simulink model "closeLoop"  (R2024a)
settings: Solver=ode45  StartTime=0.0  StopTime=100  RelTol=1e-3
values from neighbouring files (symbols this model uses):
  x = [input(1);input(2);input(3)]    [Dist_observer.m]
  y = [input(4),input(5),input(6)]'    [controller.m]
undefined symbols (not defined in the file or in its folder): initial_1, observer, saturation, z
libraries: simulink x3, slpidlib x3
settings Model: Creator=b_ant  LastModifiedBy=b_ant
settings SolverCC: ZeroCrossAlgorithm=Adaptive
settings DebuggingCC: IgnoredZcDiagnostic=none

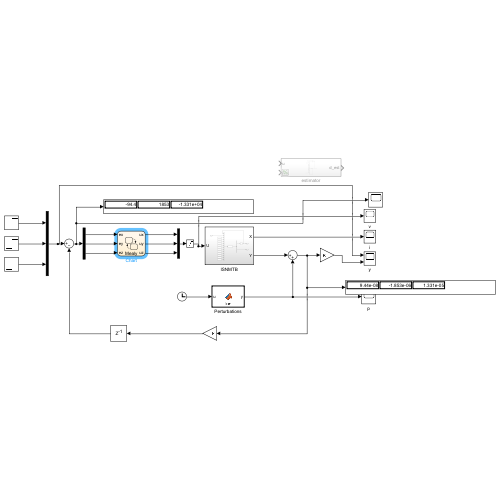
[thumbnail: Simulink's stored preview of the top-level diagram]
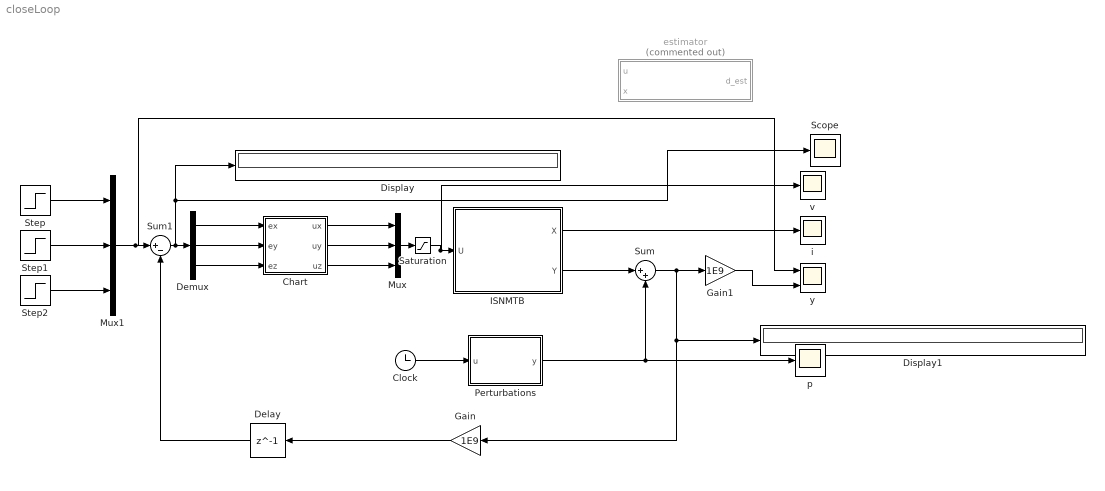
== system closeLoop ==
  Chart : Stateflow chart  TreatAsAtomicUnit=on
      settings: PortSchema="{\"entries\":[{\"content\":{\"sides\":[{\"content\":{\"connectorIds\":[\"In2\",\"In3\",\"In1\"]},\"type\":\"ConnectorPlacement.EquallySpacedRectSide\",\"uuid\":\"8b74e5db-fe86-432f-bb0a-8ff1b800d4e3\"},{\"content\":{\"connectorIds\":[\"Out2\",\"Out3\",\"Out1\"],\"side\":\"RIGHT\"},\"type\":\"ConnectorPlacement.EquallySpacedRectSide\",\"uuid\":\"0c774d5f-25b7-41fd-8d4f-dcece7db4dd0\"},{\"content\":{\"side\":\"TOP\"},\"type\":\"ConnectorPlacement.EquallySpacedRectSide\",\"uuid\":\"bb376f1f-a9bb-4d19-8a5b-9121a4c7bbab\"}]},\"type\":\"ConnectorPlacement.EquallySpacedConnector\",\"uuid\":\"4c5f25f9-8a94-4cb2-acc7-8586629943a0\"}],\"packageUris\":[\"http://schema.mathworks.com/mf0/Connector/R2020b\"],\"version\":\"1.0\"}"
  Clock : Clock
      settings: Decimation=1000
  Delay : Delay  DelayLength=1  InitialCondition=[3E4,-2E4,3E4]'  SampleTime=1E-6
  Demux : Demux  Outputs=3
  Display : Display
  Display1 : Display
  Gain : Gain  Gain=1E9
  Gain1 : Gain  Gain=1E9
  ISNMTB : Subsystem
  Mux : Mux  Inputs=3
  Mux1 : Mux  Inputs=3
  Perturbations : MATLAB Function  TreatAsAtomicUnit=on
  Saturation : Saturate  UpperLimit=[15,7,15]'  LowerLimit=[-15,-7,-15]'
  Scope : Scope
  Step : Step  After=0  SampleTime=0
  Step1 : Step  After=0  SampleTime=0
  Step2 : Step  After=0  SampleTime=0
  Sum : Sum  Inputs=|++
  Sum1 : Sum  Inputs=|+-
  estimator : Subsystem  Commented=on
  i : Scope
  p : Scope
  v : Scope
  y : Scope  NumInputPorts=2
  wires:
  ISNMTB/1(X) -> i/1
  Perturbations/1(y) -> p/1, Sum/2
  Clock/1 -> Perturbations/1(u)
  ISNMTB/2(Y) -> Sum/1
  Sum/1 -> Display1/1, Gain/1, Gain1/1
  Step/1 -> Mux1/1
  Step2/1 -> Mux1/3
  Step1/1 -> Mux1/2
  Mux1/1 -> y/1, Sum1/1
  Gain1/1 -> y/2
  Saturation/1 -> v/1, ISNMTB/1(U)
  Sum1/1 -> Scope/1, Display/1, Demux/1
  Mux/1 -> Saturation/1
  Demux/1 -> Chart/2(ex)
  Chart/2(ux) -> Mux/1
  Demux/2 -> Chart/3(ey)
  Demux/3 -> Chart/1(ez)
  Chart/1(uz) -> Mux/3
  Chart/3(uy) -> Mux/2
  Delay/1 -> Sum1/2
  Gain/1 -> Delay/1

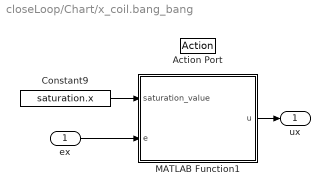
== system closeLoop/Chart/x_coil.bang_bang ==
  ex : Inport
  Action Port : ActionPort
      settings: CopyFcn=Stateflow.SLINSF.SimulinkMan.removeBlockPreDeleteFcn  PreDeleteFcn=Stateflow.SLINSF.SimulinkMan.unsafePredeleteFcn
  Constant9 : Constant  Value=saturation.x
  MATLAB Function1 : MATLAB Function  TreatAsAtomicUnit=on
  ux : Outport
  wires:
  MATLAB Function1/1(u) -> ux/1
  ex/1 -> MATLAB Function1/2(e)
  Constant9/1 -> MATLAB Function1/1(saturation_value)

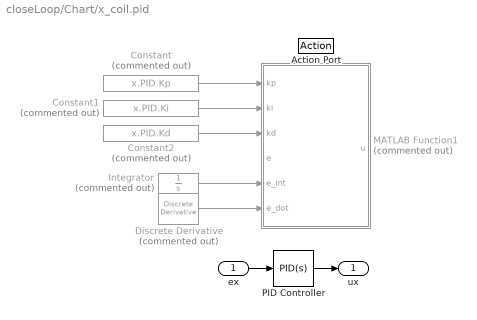
== system closeLoop/Chart/x_coil.pid ==
  ex : Inport
  Action Port : ActionPort
      settings: CopyFcn=Stateflow.SLINSF.SimulinkMan.removeBlockPreDeleteFcn  PreDeleteFcn=Stateflow.SLINSF.SimulinkMan.unsafePredeleteFcn
  Constant : Constant  Commented=on  Value=x.PID.Kp
  Constant1 : Constant  Commented=on  Value=x.PID.Ki
  Constant2 : Constant  Commented=on  Value=x.PID.Kd
  Discrete Derivative : simulink/Discrete/Discrete Derivative  Commented=on  gainval=1.0  ICPrevScaledInput=0.0  OutMin=[]  OutMax=[]  OutDataType=fixdt(1, 16)  OutScaling=2^-10  DoSatur=off
  Integrator : Integrator  Commented=on
  MATLAB Function1 : MATLAB Function  Commented=on  TreatAsAtomicUnit=on
  PID Controller : slpidlib/PID Controller  Controller=PID  Form=Parallel  TimeDomain=Continuous-time  UseExternalTs=off  SampleTime=-1  IntegratorMethod=Forward Euler  FilterMethod=Forward Euler  ControllerParametersSource=internal  P=x.PID.Kp  I=x.PID.Ki  UseKiTs=off  D=x.PID.Kd  UseExternalDerivativeSource=off  N=100  UseFilter=on  TunerSelectOption=Transfer Function Based (PID Tuner App)  InitialConditionSource=internal  InitialConditionForIntegrator=0  InitialConditionForFilter=0  DifferentiatorICPrevScaledInput=0  ExternalReset=none  TrackingMode=off  Kt=1  LimitOutput=off  SatLimitsSource=internal  UpperSaturationLimit=inf  LowerSaturationLimit=-inf  LinearizeAsGain=on  AntiWindupMode=none  Kb=1  LimitIntegrator=off  UpperIntegratorSaturationLimit=inf  LowerIntegratorSaturationLimit=-inf  POutMin=[]  POutMax=[]  IOutMin=[]  IOutMax=[]  DOutMin=[]  DOutMax=[]  NOutMin=[]  NOutMax=[]  SumOutMin=[]  SumOutMax=[]  SaturationOutMin=[]  SaturationOutMax=[]  PParamMin=[]  PParamMax=[]  IParamMin=[]  IParamMax=[]  DParamMin=[]  DParamMax=[]  NParamMin=[]  NParamMax=[]  KbParamMin=[]  KbParamMax=[]  KtParamMin=[]  KtParamMax=[]  KbOutMin=[]  KbOutMax=[]  KtOutMin=[]  KtOutMax=[]  IntegratorOutMin=[]  IntegratorOutMax=[]  FilterOutMin=[]  FilterOutMax=[]  SumI1OutMin=[]  SumI1OutMax=[]  SumI2OutMin=[]  SumI2OutMax=[]  SumI3OutMin=[]  SumI3OutMax=[]  SumI4OutMin=[]  SumI4OutMax=[]  SumDOutMin=[]  SumDOutMax=[]  DifferentiatorOutMin=[]  DifferentiatorOutMax=[]  FilterDiffOutCoefMin=[]  FilterDiffOutCoefMax=[]  ReciprocalOutMin=[]  ReciprocalOutMax=[]  SumDenOutMin=[]  SumDenOutMax=[]  SumNumOutMin=[]  SumNumOutMax=[]  DivideOutMin=[]  DivideOutMax=[]  UdiffTsProdOutMin=[]  UdiffTsProdOutMax=[]  NTsProdOutMin=[]  NTsProdOutMax=[]  UintegralTsProdOutMin=[]  UintegralTsProdOutMax=[]  UngainTsProdOutMin=[]  UngainTsProdOutMax=[]  ClampingZeroOutDataTypeStr=Inherit: Inherit via back propagation  ClampingZeroOutMin=[]  ClampingZeroOutMax=[]  FilterDenConstantOutDataTypeStr=Inherit: Inherit via back propagation  FilterDenConstantOutMin=[]  FilterDenConstantOutMax=[]  PCopyOutDataTypeStr=Inherit: Inherit via back propagation  PCopyOutMin=[]  PCopyOutMax=[]  NCopyOutDataTypeStr=Inherit: Inherit via back propagation  NCopyOutMin=[]  NCopyOutMax=[]  IntegratorContinuousStateAttributes=''  IntegratorStateMustResolveToSignalObject=off  IntegratorRTWStateStorageClass=Auto  FilterContinuousStateAttributes=''  FilterStateMustResolveToSignalObject=off  FilterRTWStateStorageClass=Auto  ParallelPVariant=InternalParameters  IdealPVariant=Disabled  IVariant=InternalParameters  DVariant=InternalParameters  IntegratorVariant=Continuous  SatVariant=Disabled  AWVariant=Passthrough  PCopyVariant=Disabled  TRVariant=Disabled  FdbkBlocksVariant=Forward  IdealPFdbkVariant=Disabled  SatFdbkVariant=Disabled  DerivativeFilterVariant=ContFilter  NVariant=InternalParameters  NCopyVariant=Disabled  FilterICVariant=InternalICsFilter  IntegratorICVariant=InternalICs  ExternalResetVariant=Disabled  TRSumVariant=Passthrough  SumFdbkVariant=Disabled  SumVariant=Sum_PID  TsampFilterVariant=InternalTs  TsampNgainVariant=Passthrough  TsampIntegralVariant=Disabled_SignalSpec  ExternalSaturationOutDataTypeStr=Inherit: Same as second input  DerivativeSourceVariant=ErrorSignal
  ux : Outport
  wires:
  Integrator/1 -> MATLAB Function1/5(e_int)
  Constant1/1 -> MATLAB Function1/2(ki)
  Constant2/1 -> MATLAB Function1/3(kd)
  Discrete Derivative/1 -> MATLAB Function1/6(e_dot)
  Constant/1 -> MATLAB Function1/1(kp)
  PID Controller/1 -> ux/1
  ex/1 -> PID Controller/1

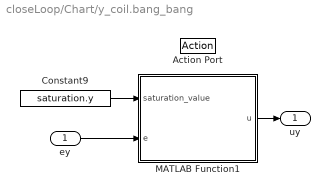
== system closeLoop/Chart/y_coil.bang_bang ==
  ey : Inport
  Action Port : ActionPort
      settings: CopyFcn=Stateflow.SLINSF.SimulinkMan.removeBlockPreDeleteFcn  PreDeleteFcn=Stateflow.SLINSF.SimulinkMan.unsafePredeleteFcn
  Constant9 : Constant  Value=saturation.y
  MATLAB Function1 : MATLAB Function  TreatAsAtomicUnit=on
  uy : Outport
  wires:
  MATLAB Function1/1(u) -> uy/1
  ey/1 -> MATLAB Function1/2(e)
  Constant9/1 -> MATLAB Function1/1(saturation_value)

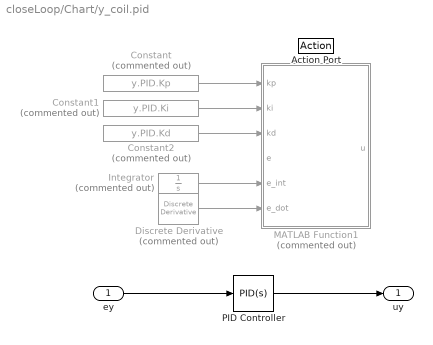
== system closeLoop/Chart/y_coil.pid ==
  ey : Inport
  Action Port : ActionPort
      settings: CopyFcn=Stateflow.SLINSF.SimulinkMan.removeBlockPreDeleteFcn  PreDeleteFcn=Stateflow.SLINSF.SimulinkMan.unsafePredeleteFcn
  Constant : Constant  Commented=on  Value=y.PID.Kp
  Constant1 : Constant  Commented=on  Value=y.PID.Ki
  Constant2 : Constant  Commented=on  Value=y.PID.Kd
  Discrete Derivative : simulink/Discrete/Discrete Derivative  Commented=on  gainval=1.0  ICPrevScaledInput=0.0  OutMin=[]  OutMax=[]  OutDataType=fixdt(1, 16)  OutScaling=2^-10  DoSatur=off
  Integrator : Integrator  Commented=on
  MATLAB Function1 : MATLAB Function  Commented=on  TreatAsAtomicUnit=on
  PID Controller : slpidlib/PID Controller  Controller=PID  Form=Parallel  TimeDomain=Continuous-time  UseExternalTs=off  SampleTime=-1  IntegratorMethod=Forward Euler  FilterMethod=Forward Euler  ControllerParametersSource=internal  P=y.PID.Kp  I=y.PID.Ki  UseKiTs=off  D=y.PID.Kd  UseExternalDerivativeSource=off  N=100  UseFilter=on  TunerSelectOption=Transfer Function Based (PID Tuner App)  InitialConditionSource=internal  InitialConditionForIntegrator=0  InitialConditionForFilter=0  DifferentiatorICPrevScaledInput=0  ExternalReset=none  TrackingMode=off  Kt=1  LimitOutput=off  SatLimitsSource=internal  UpperSaturationLimit=inf  LowerSaturationLimit=-inf  LinearizeAsGain=on  AntiWindupMode=none  Kb=1  LimitIntegrator=off  UpperIntegratorSaturationLimit=inf  LowerIntegratorSaturationLimit=-inf  POutMin=[]  POutMax=[]  IOutMin=[]  IOutMax=[]  DOutMin=[]  DOutMax=[]  NOutMin=[]  NOutMax=[]  SumOutMin=[]  SumOutMax=[]  SaturationOutMin=[]  SaturationOutMax=[]  PParamMin=[]  PParamMax=[]  IParamMin=[]  IParamMax=[]  DParamMin=[]  DParamMax=[]  NParamMin=[]  NParamMax=[]  KbParamMin=[]  KbParamMax=[]  KtParamMin=[]  KtParamMax=[]  KbOutMin=[]  KbOutMax=[]  KtOutMin=[]  KtOutMax=[]  IntegratorOutMin=[]  IntegratorOutMax=[]  FilterOutMin=[]  FilterOutMax=[]  SumI1OutMin=[]  SumI1OutMax=[]  SumI2OutMin=[]  SumI2OutMax=[]  SumI3OutMin=[]  SumI3OutMax=[]  SumI4OutMin=[]  SumI4OutMax=[]  SumDOutMin=[]  SumDOutMax=[]  DifferentiatorOutMin=[]  DifferentiatorOutMax=[]  FilterDiffOutCoefMin=[]  FilterDiffOutCoefMax=[]  ReciprocalOutMin=[]  ReciprocalOutMax=[]  SumDenOutMin=[]  SumDenOutMax=[]  SumNumOutMin=[]  SumNumOutMax=[]  DivideOutMin=[]  DivideOutMax=[]  UdiffTsProdOutMin=[]  UdiffTsProdOutMax=[]  NTsProdOutMin=[]  NTsProdOutMax=[]  UintegralTsProdOutMin=[]  UintegralTsProdOutMax=[]  UngainTsProdOutMin=[]  UngainTsProdOutMax=[]  ClampingZeroOutDataTypeStr=Inherit: Inherit via back propagation  ClampingZeroOutMin=[]  ClampingZeroOutMax=[]  FilterDenConstantOutDataTypeStr=Inherit: Inherit via back propagation  FilterDenConstantOutMin=[]  FilterDenConstantOutMax=[]  PCopyOutDataTypeStr=Inherit: Inherit via back propagation  PCopyOutMin=[]  PCopyOutMax=[]  NCopyOutDataTypeStr=Inherit: Inherit via back propagation  NCopyOutMin=[]  NCopyOutMax=[]  IntegratorContinuousStateAttributes=''  IntegratorStateMustResolveToSignalObject=off  IntegratorRTWStateStorageClass=Auto  FilterContinuousStateAttributes=''  FilterStateMustResolveToSignalObject=off  FilterRTWStateStorageClass=Auto  ParallelPVariant=InternalParameters  IdealPVariant=Disabled  IVariant=InternalParameters  DVariant=InternalParameters  IntegratorVariant=Continuous  SatVariant=Disabled  AWVariant=Passthrough  PCopyVariant=Disabled  TRVariant=Disabled  FdbkBlocksVariant=Forward  IdealPFdbkVariant=Disabled  SatFdbkVariant=Disabled  DerivativeFilterVariant=ContFilter  NVariant=InternalParameters  NCopyVariant=Disabled  FilterICVariant=InternalICsFilter  IntegratorICVariant=InternalICs  ExternalResetVariant=Disabled  TRSumVariant=Passthrough  SumFdbkVariant=Disabled  SumVariant=Sum_PID  TsampFilterVariant=InternalTs  TsampNgainVariant=Passthrough  TsampIntegralVariant=Disabled_SignalSpec  ExternalSaturationOutDataTypeStr=Inherit: Same as second input  DerivativeSourceVariant=ErrorSignal
  uy : Outport
  wires:
  Integrator/1 -> MATLAB Function1/5(e_int)
  Constant1/1 -> MATLAB Function1/2(ki)
  Constant2/1 -> MATLAB Function1/3(kd)
  Discrete Derivative/1 -> MATLAB Function1/6(e_dot)
  Constant/1 -> MATLAB Function1/1(kp)
  ey/1 -> PID Controller/1
  PID Controller/1 -> uy/1

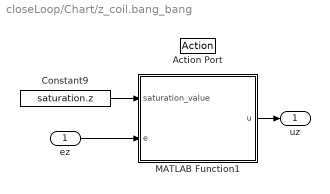
== system closeLoop/Chart/z_coil.bang_bang ==
  ez : Inport
  Action Port : ActionPort
      settings: CopyFcn=Stateflow.SLINSF.SimulinkMan.removeBlockPreDeleteFcn  PreDeleteFcn=Stateflow.SLINSF.SimulinkMan.unsafePredeleteFcn
  Constant9 : Constant  Value=saturation.z
  MATLAB Function1 : MATLAB Function  TreatAsAtomicUnit=on
  uz : Outport
  wires:
  MATLAB Function1/1(u) -> uz/1
  ez/1 -> MATLAB Function1/2(e)
  Constant9/1 -> MATLAB Function1/1(saturation_value)

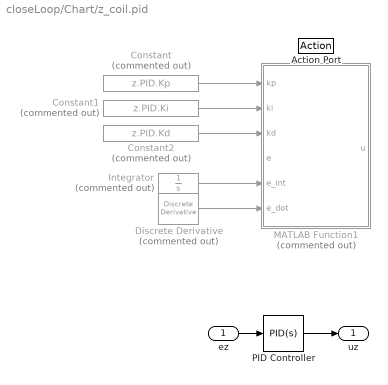
== system closeLoop/Chart/z_coil.pid ==
  ez : Inport
  Action Port : ActionPort
      settings: CopyFcn=Stateflow.SLINSF.SimulinkMan.removeBlockPreDeleteFcn  PreDeleteFcn=Stateflow.SLINSF.SimulinkMan.unsafePredeleteFcn
  Constant : Constant  Commented=on  Value=z.PID.Kp
  Constant1 : Constant  Commented=on  Value=z.PID.Ki
  Constant2 : Constant  Commented=on  Value=z.PID.Kd
  Discrete Derivative : simulink/Discrete/Discrete Derivative  Commented=on  gainval=1.0  ICPrevScaledInput=0.0  OutMin=[]  OutMax=[]  OutDataType=fixdt(1, 16)  OutScaling=2^-10  DoSatur=off
  Integrator : Integrator  Commented=on
  MATLAB Function1 : MATLAB Function  Commented=on  TreatAsAtomicUnit=on
  PID Controller : slpidlib/PID Controller  Controller=PID  Form=Parallel  TimeDomain=Continuous-time  UseExternalTs=off  SampleTime=-1  IntegratorMethod=Forward Euler  FilterMethod=Forward Euler  ControllerParametersSource=internal  P=z.PID.Kp  I=z.PID.Ki  UseKiTs=off  D=z.PID.Kd  UseExternalDerivativeSource=off  N=100  UseFilter=on  TunerSelectOption=Transfer Function Based (PID Tuner App)  InitialConditionSource=internal  InitialConditionForIntegrator=0  InitialConditionForFilter=0  DifferentiatorICPrevScaledInput=0  ExternalReset=none  TrackingMode=off  Kt=1  LimitOutput=off  SatLimitsSource=internal  UpperSaturationLimit=inf  LowerSaturationLimit=-inf  LinearizeAsGain=on  AntiWindupMode=none  Kb=1  LimitIntegrator=off  UpperIntegratorSaturationLimit=inf  LowerIntegratorSaturationLimit=-inf  POutMin=[]  POutMax=[]  IOutMin=[]  IOutMax=[]  DOutMin=[]  DOutMax=[]  NOutMin=[]  NOutMax=[]  SumOutMin=[]  SumOutMax=[]  SaturationOutMin=[]  SaturationOutMax=[]  PParamMin=[]  PParamMax=[]  IParamMin=[]  IParamMax=[]  DParamMin=[]  DParamMax=[]  NParamMin=[]  NParamMax=[]  KbParamMin=[]  KbParamMax=[]  KtParamMin=[]  KtParamMax=[]  KbOutMin=[]  KbOutMax=[]  KtOutMin=[]  KtOutMax=[]  IntegratorOutMin=[]  IntegratorOutMax=[]  FilterOutMin=[]  FilterOutMax=[]  SumI1OutMin=[]  SumI1OutMax=[]  SumI2OutMin=[]  SumI2OutMax=[]  SumI3OutMin=[]  SumI3OutMax=[]  SumI4OutMin=[]  SumI4OutMax=[]  SumDOutMin=[]  SumDOutMax=[]  DifferentiatorOutMin=[]  DifferentiatorOutMax=[]  FilterDiffOutCoefMin=[]  FilterDiffOutCoefMax=[]  ReciprocalOutMin=[]  ReciprocalOutMax=[]  SumDenOutMin=[]  SumDenOutMax=[]  SumNumOutMin=[]  SumNumOutMax=[]  DivideOutMin=[]  DivideOutMax=[]  UdiffTsProdOutMin=[]  UdiffTsProdOutMax=[]  NTsProdOutMin=[]  NTsProdOutMax=[]  UintegralTsProdOutMin=[]  UintegralTsProdOutMax=[]  UngainTsProdOutMin=[]  UngainTsProdOutMax=[]  ClampingZeroOutDataTypeStr=Inherit: Inherit via back propagation  ClampingZeroOutMin=[]  ClampingZeroOutMax=[]  FilterDenConstantOutDataTypeStr=Inherit: Inherit via back propagation  FilterDenConstantOutMin=[]  FilterDenConstantOutMax=[]  PCopyOutDataTypeStr=Inherit: Inherit via back propagation  PCopyOutMin=[]  PCopyOutMax=[]  NCopyOutDataTypeStr=Inherit: Inherit via back propagation  NCopyOutMin=[]  NCopyOutMax=[]  IntegratorContinuousStateAttributes=''  IntegratorStateMustResolveToSignalObject=off  IntegratorRTWStateStorageClass=Auto  FilterContinuousStateAttributes=''  FilterStateMustResolveToSignalObject=off  FilterRTWStateStorageClass=Auto  ParallelPVariant=InternalParameters  IdealPVariant=Disabled  IVariant=InternalParameters  DVariant=InternalParameters  IntegratorVariant=Continuous  SatVariant=Disabled  AWVariant=Passthrough  PCopyVariant=Disabled  TRVariant=Disabled  FdbkBlocksVariant=Forward  IdealPFdbkVariant=Disabled  SatFdbkVariant=Disabled  DerivativeFilterVariant=ContFilter  NVariant=InternalParameters  NCopyVariant=Disabled  FilterICVariant=InternalICsFilter  IntegratorICVariant=InternalICs  ExternalResetVariant=Disabled  TRSumVariant=Passthrough  SumFdbkVariant=Disabled  SumVariant=Sum_PID  TsampFilterVariant=InternalTs  TsampNgainVariant=Passthrough  TsampIntegralVariant=Disabled_SignalSpec  ExternalSaturationOutDataTypeStr=Inherit: Same as second input  DerivativeSourceVariant=ErrorSignal
  uz : Outport
  wires:
  Integrator/1 -> MATLAB Function1/5(e_int)
  Constant1/1 -> MATLAB Function1/2(ki)
  Constant2/1 -> MATLAB Function1/3(kd)
  Discrete Derivative/1 -> MATLAB Function1/6(e_dot)
  Constant/1 -> MATLAB Function1/1(kp)
  ez/1 -> PID Controller/1
  PID Controller/1 -> uz/1

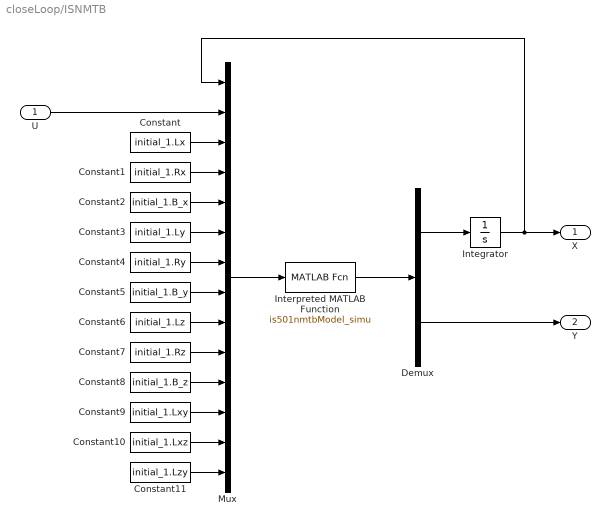
== system closeLoop/ISNMTB ==
  U : Inport
  Constant : Constant  Value=initial_1.Lx
  Constant1 : Constant  Value=initial_1.Rx
  Constant10 : Constant  Value=initial_1.Lxz
  Constant11 : Constant  Value=initial_1.Lzy
  Constant2 : Constant  Value=initial_1.B_x
  Constant3 : Constant  Value=initial_1.Ly
  Constant4 : Constant  Value=initial_1.Ry
  Constant5 : Constant  Value=initial_1.B_y
  Constant6 : Constant  Value=initial_1.Lz
  Constant7 : Constant  Value=initial_1.Rz
  Constant8 : Constant  Value=initial_1.B_z
  Constant9 : Constant  Value=initial_1.Lxy
  Demux : Demux  Outputs=2
  Integrator : Integrator  InitialCondition=[0,0,0]
  Interpreted MATLAB Function : MATLABFcn  MATLABFcn=is501nmtbModel_simu  OutputDimensions=6
  Mux : Mux  Inputs=14
  X : Outport
  Y : Outport  Port=2
  wires:
  Constant2/1 -> Mux/5
  Constant/1 -> Mux/3
  Demux/1 -> Integrator/1
  Interpreted MATLAB Function/1 -> Demux/1
  Constant9/1 -> Mux/12
  Constant5/1 -> Mux/8
  Constant3/1 -> Mux/6
  Constant1/1 -> Mux/4
  Integrator/1 -> X/1, Mux/1
  Mux/1 -> Interpreted MATLAB Function/1
  Constant10/1 -> Mux/13
  Constant7/1 -> Mux/10
  Constant11/1 -> Mux/14
  Constant4/1 -> Mux/7
  Constant8/1 -> Mux/11
  Constant6/1 -> Mux/9
  U/1 -> Mux/2
  Demux/2 -> Y/1

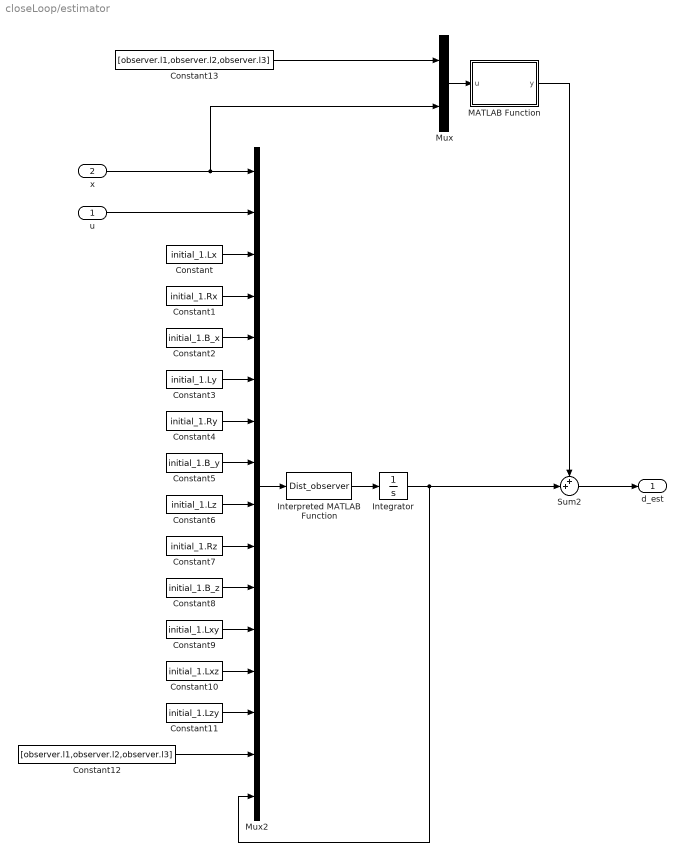
== system closeLoop/estimator ==
  u : Inport
  x : Inport  Port=2
  Constant : Constant  Value=initial_1.Lx
  Constant1 : Constant  Value=initial_1.Rx
  Constant10 : Constant  Value=initial_1.Lxz
  Constant11 : Constant  Value=initial_1.Lzy
  Constant12 : Constant  Value=[observer.l1,observer.l2,observer.l3]
  Constant13 : Constant  Value=[observer.l1,observer.l2,observer.l3]
  Constant2 : Constant  Value=initial_1.B_x
  Constant3 : Constant  Value=initial_1.Ly
  Constant4 : Constant  Value=initial_1.Ry
  Constant5 : Constant  Value=initial_1.B_y
  Constant6 : Constant  Value=initial_1.Lz
  Constant7 : Constant  Value=initial_1.Rz
  Constant8 : Constant  Value=initial_1.B_z
  Constant9 : Constant  Value=initial_1.Lxy
  Integrator : Integrator  InitialCondition=[0,0,0]
  Interpreted MATLAB Function : MATLABFcn  MATLABFcn=Dist_observer
  MATLAB Function : MATLAB Function  TreatAsAtomicUnit=on
  Mux : Mux  Inputs=2
  Mux2 : Mux  Inputs=16
  Sum2 : Sum  Inputs=++|
  d_est : Outport
  wires:
  Constant6/1 -> Mux2/9
  MATLAB Function/1(y) -> Sum2/1
  x/1 -> Mux/2, Mux2/1
  Constant10/1 -> Mux2/13
  Integrator/1 -> Sum2/2, Mux2/16
  Interpreted MATLAB Function/1 -> Integrator/1
  Constant2/1 -> Mux2/5
  Constant4/1 -> Mux2/7
  Constant7/1 -> Mux2/10
  Mux2/1 -> Interpreted MATLAB Function/1
  Constant11/1 -> Mux2/14
  Constant8/1 -> Mux2/11
  Constant1/1 -> Mux2/4
  Constant3/1 -> Mux2/6
  Constant/1 -> Mux2/3
  Constant9/1 -> Mux2/12
  Constant5/1 -> Mux2/8
  Constant12/1 -> Mux2/15
  u/1 -> Mux2/2
  Sum2/1 -> d_est/1
  Constant13/1 -> Mux/1
  Mux/1 -> MATLAB Function/1(u)

== matlab function closeLoop/Chart/x_coil.bang_bang/MATLAB Function1 ==
  data: saturation_value input; u output; e input
function u  = bangbang(saturation_value,e) 
        u = saturation_value*sign(e);
end

== matlab function closeLoop/Chart/y_coil.bang_bang/MATLAB Function1 ==
  data: saturation_value input; u output; e input
function u  = bangbang(saturation_value,e) 
        u = saturation_value*sign(e);
end

== matlab function closeLoop/Chart/y_coil.pid/MATLAB Function1 ==
  data: u output; kp input; ki input; kd input; e input; e_int input; e_dot input
function u  = pid_controller(kp, ki, kd, e, e_int, e_dot) 
    u=kp*e+ki*e_int+kd*e_dot;
end

== matlab function closeLoop/Chart/z_coil.pid/MATLAB Function1 ==
  data: u output; kp input; ki input; kd input; e input; e_int input; e_dot input
function u  = pid_controller(kp, ki, kd, e, e_int, e_dot) 
    u=kp*e+ki*e_int+kd*e_dot;
end

== matlab function closeLoop/Chart/z_coil.bang_bang/MATLAB Function1 ==
  data: saturation_value input; u output; e input
function u  = bangbang(saturation_value,e) 
        u = saturation_value*sign(e);
end

== matlab function closeLoop/estimator/MATLAB Function ==
  data: u input; y output
function y = fcn(u)
l = diag([u(1),u(2),u(3)]);
x = [u(4);u(5);u(6)];

y = l*x;
end

== matlab function closeLoop/Perturbations ==
  data: u input; y output
function y = fcn(u)
y= [2.522*sin(2*pi*4.788E-3*u)+3.249E04;
   -5.174*sin(2*pi*7.481E-3*u)-2.265E04;
    3.359*sin(2*pi*8.378E-3*u)+3.655E04]*1E-9;
end

== stateflow chart closeLoop/Chart ==
  settings: updateMethod=CONTINUOUS  sampleTime=1E-3  stateMachineType=MEALY_MACHINE
  state x_coil [parallel]
    settings: executionOrder=1
    state bang_bang
    state pid
    (default) -> x_coil.bang_bang
    x_coil.bang_bang -> x_coil.pid : [abs(ex)<100]
  state y_coil [parallel]
    settings: executionOrder=2
    state bang_bang
    state pid
    (default) -> y_coil.bang_bang
    y_coil.bang_bang -> y_coil.pid : [abs(ey)<100]
  state z_coil [parallel]
    settings: executionOrder=3
    state bang_bang
    state pid
    (default) -> z_coil.bang_bang
    z_coil.bang_bang -> z_coil.pid : [abs(ez)<100]
  data: sf_internal_action_state_placeholder_data local double size=1 =0; sf_internal_action_state_placeholder_data local double size=1 =0; sf_internal_action_state_placeholder_data local double size=1 =0; sf_internal_action_state_placeholder_data local double size=1 =0; sf_internal_action_state_placeholder_data local double size=1 =0; sf_internal_action_state_placeholder_data local double size=1 =0; ez input; uz output; ex input; ux output; ey input; uy output

== matlab function closeLoop/Chart/x_coil.pid/MATLAB Function1 ==
  data: u output; kp input; ki input; kd input; e input; e_int input; e_dot input
function u  = pid_controller(kp, ki, kd, e, e_int, e_dot) 
    u=kp*e+ki*e_int+kd*e_dot;
end
